simulink model "amo"  (R2022b)
settings: Solver=VariableStepAuto  StartTime=0.0  StopTime=20  RelTol=1e-3
values from neighbouring files (symbols this model uses):
  K = real(-1 / (L(s0) * C(s0)))    [controller.m]
undefined symbols (not defined in the file or in its folder): A, B, x_initial, x_ref
settings Model: Creator=Sina  LastModifiedBy=JNemune
settings OptimizationCC: ReuseModelBlockBuffer=on
settings RTWCC: GPUComputeCapability=5.0

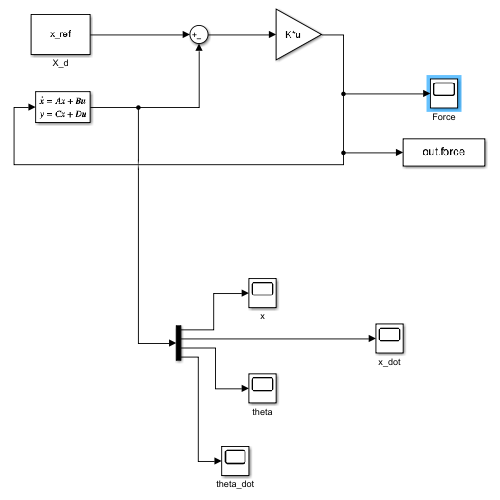
[thumbnail: Simulink's stored preview of the top-level diagram]
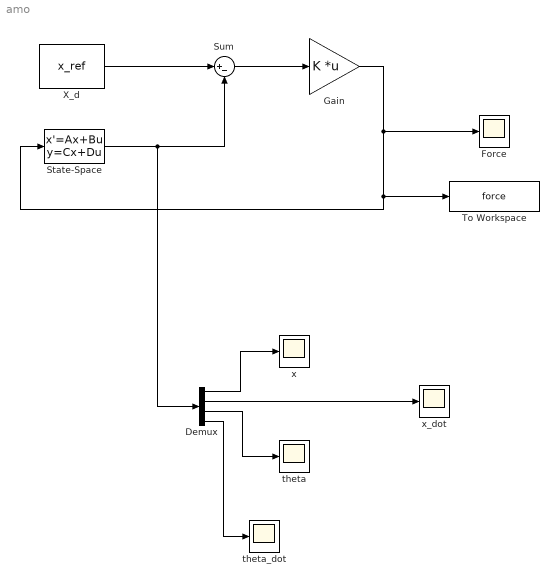
== system amo ==
  Demux : Demux
  Force : Scope
  Gain : Gain  Gain=K  Multiplication=Matrix(K*u)
  State-Space : StateSpace  A=A  B=B  C=eye(4)  D=zeros(4,1)  InitialCondition=x_initial
  Sum : Sum  Inputs=|+-
  To Workspace : ToWorkspace  VariableName=force  SaveFormat=Timeseries  SampleTime=-1
  X_d : Constant  Value=x_ref
  theta : Scope
  theta_dot : Scope
  x : Scope
  x_dot : Scope
  wires:
  X_d/1 -> Sum/1
  State-Space/1 -> Demux/1, Sum/2
  Sum/1 -> Gain/1
  Gain/1 -> To Workspace/1, State-Space/1, Force/1
  Demux/1 -> x/1
  Demux/3 -> theta/1
  Demux/2 -> x_dot/1
  Demux/4 -> theta_dot/1
